simulink model "sl_mobile_vs"  (Simulink 9.1)
settings: Solver=ode45  StartTime=0.0  StopTime=10  RelTol=1e-3  EnableMultiTasking=on
InitFcn:
  | camera = CentralCamera('default', 'name', 'mobile_vs', 'focal', 0.002);
  | T_vc = transl(0.2, 0.1, 0.3)*troty(pi/2)*trotz(-pi/2); %*trotx(-pi/4);
  | P = [0 0; 1 -1; 2 2];
  | pstar = camera.project(P, 'Tcam', transl(-2, 0, 0)*T_vc);
undefined symbols (not defined in the file or in its folder): cond, DiscIntNeverNeededParam, tose2, tose3
libraries: roblocks x2, simulink x1
settings Model: Creator=pic  LastModifiedBy=83789  ExtModeTrigMode=oneshot  ExtModeArmWhenConnect=off
settings DataIOCC: SaveFormat=Structure  SignalLoggingSaveFormat=ModelDataLogs  ReturnWorkspaceOutputs=on
settings OptimizationCC: BlockReduction=off  BooleanDataType=off  ExpressionDepthLimit=2147483647  InitFltsAndDblsToZero=on
settings DebuggingCC: SaveWithParameterizedLinksMsg=none  SignalResolutionControl=TryResolveAllWithWarning  MultiTaskDSMMsg=warning  MultiTaskCondExecSysMsg=none  FcnCallInpInsideContextMsg=warning  StateNameClashWarn=warning
settings HardwareCC: TargetUnknown=on
settings GRTTargetCC: ModelReferenceCompliant=off  CompOptLevelCompliant=off  GeneratePreprocessorConditionals=Disable all  MatFileLogging=off
settings ConfigComp: CovSFcnEnable=off

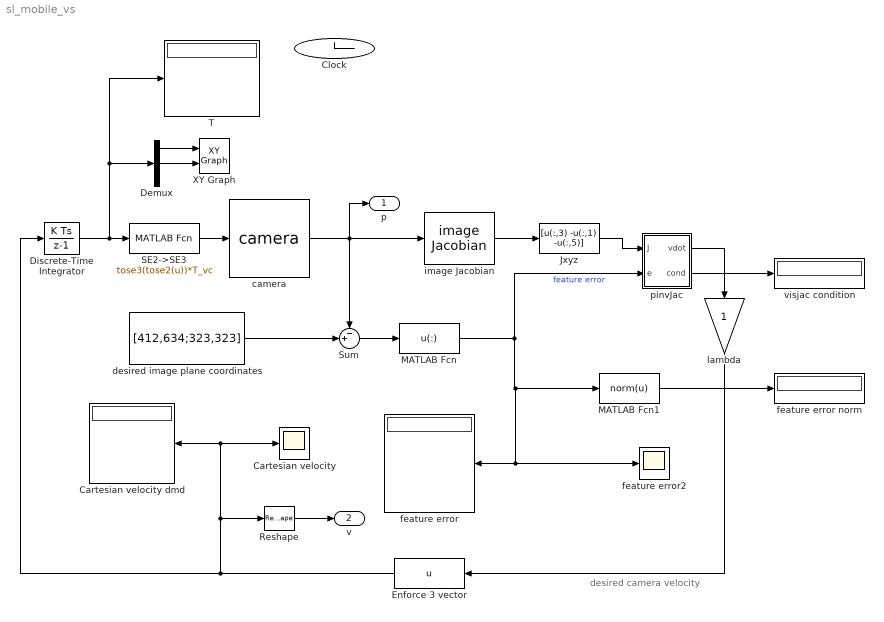
== system sl_mobile_vs ==
  note: desired camera velocity
  Cartesian velocity : Scope
  Cartesian velocity dmd : Display
      settings: Format=short_e
  Clock : Clock
  Demux : Demux  Outputs=3
  Discrete-Time Integrator : DiscreteIntegrator  InitialCondition=[-8 2 0.3]'  SampleTime=0.02  ICPrevOutput=DiscIntNeverNeededParam  ICPrevScaledInput=DiscIntNeverNeededParam
  Enforce 3 vector : MATLABFcn  MATLABFcn=u  OutputDimensions=3  Output1D=off
  Jxyz : MATLABFcn  MATLABFcn=[u(:,3) -u(:,1) -u(:,5)]  Output1D=off
  MATLAB Fcn : MATLABFcn  MATLABFcn=u(:)  Output1D=off
  MATLAB Fcn1 : MATLABFcn  MATLABFcn=norm(u)
  Reshape : Reshape  OutputDimensionality=Customize  OutputDimensions=3
  SE2->SE3 : MATLABFcn  MATLABFcn=tose3(tose2(u))*T_vc  Output1D=off
  Sum : Sum  Inputs=-+|  SaturateOnIntegerOverflow=on  InputSameDT=on  OutDataTypeStr=Inherit: Same as first input
  T : Display
  XY Graph : simulink/Sinks/XY Graph  xmin=-10  xmax=10  ymin=-10  ymax=10  st=-1
  camera : roblocks/Vision/camera  cam=camera  points=P
      link override MATLAB Fcn: MATLABFcn=cam.plot(points, 'pose', u)
  desired image plane coordinates : Constant  Value=[412,634;323,323]  VectorParams1D=off
  feature error : Display
      settings: Format=bank
  feature error norm : Display
  feature error2 : Scope
  image Jacobian : roblocks/Vision/image Jacobian  cam=camera  z=2
  lambda : Gain  SaturateOnIntegerOverflow=on  OutDataTypeStr=Inherit: Same as input  ParamDataTypeStr=Inherit: Same as input
  pinvJac : Subsystem
  visjac condition : Display
  p : Outport
  v : Outport  Port=2
  wires:
  camera/1 -> Sum/1, p/1, image Jacobian/1
  Sum/1 -> MATLAB Fcn/1
  desired image plane coordinates/1 -> Sum/2
  MATLAB Fcn/1 -> pinvJac/2(e), MATLAB Fcn1/1, feature error2/1, feature error/1  "feature error"
  MATLAB Fcn1/1 -> feature error norm/1
  Discrete-Time Integrator/1 -> SE2->SE3/1, T/1, Demux/1
  image Jacobian/1 -> Jxyz/1
  Jxyz/1 -> pinvJac/1(J)
  SE2->SE3/1 -> camera/1
  Demux/1 -> XY Graph/1
  Demux/2 -> XY Graph/2
  Reshape/1 -> v/1
  lambda/1 -> Enforce 3 vector/1
  Enforce 3 vector/1 -> Cartesian velocity dmd/1, Cartesian velocity/1, Reshape/1, Discrete-Time Integrator/1
  pinvJac/1(vdot) -> lambda/1
  pinvJac/2(cond) -> visjac condition/1

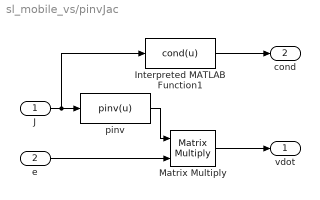
== system sl_mobile_vs/pinvJac ==
  J : Inport
  e : Inport  Port=2
  Interpreted MATLAB Function1 : MATLABFcn  MATLABFcn=cond(u)  Output1D=off
  Matrix Multiply : Product  Multiplication=Matrix(*)
  pinv : MATLABFcn  MATLABFcn=pinv(u)  Output1D=off
  vdot : Outport
  cond : Outport  Port=2
  wires:
  J/1 -> Interpreted MATLAB Function1/1, pinv/1
  e/1 -> Matrix Multiply/2
  pinv/1 -> Matrix Multiply/1
  Matrix Multiply/1 -> vdot/1
  Interpreted MATLAB Function1/1 -> cond/1
